simulink model "copied"  (R2019a)
settings: Solver=VariableStepAuto  StartTime=0.0  StopTime=10.0  RelTol=1e-3
libraries: vexarmcortexlib x21, vexcommonlib x3
settings Model: Creator=hsstudent  LastModifiedBy=hsstudent

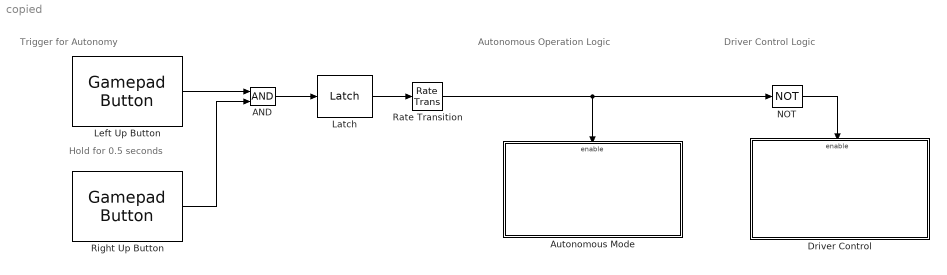
== system copied ==
  note: Autonomous Operation Logic
  note: Trigger for Autonomy
  note: Hold for 0.5 seconds
  note: Driver Control Logic
  AND : Logic  IconShape=distinctive  AllPortsSameDT=off  OutDataTypeStr=boolean
  Autonomous Mode : Subsystem
  Driver Control : Subsystem  TreatAsAtomicUnit=on
  Latch : vexcommonlib/Latch  output0=off  BlockPlatform=vexarmcortex
      settings: SourceProductName=Simulink Coder Support Package for ARM Cortex-based VEX Microcontroller  SourceProductBaseCode=EC_VEX_MICRO
  Left Up Button : vexarmcortexlib/Gamepad/Gamepad Button  joystick=1  chan=7  button56=Down  button78=Up  SimulationIn=off  SampleTime=0.5
      settings: SourceProductName=Simulink Coder Support Package for ARM Cortex-based VEX Microcontroller  SourceProductBaseCode=EC_VEX_MICRO
  NOT : Logic  Operator=NOT  IconShape=distinctive  AllPortsSameDT=off  OutDataTypeStr=boolean
  Rate Transition : RateTransition
  Right Up Button : vexarmcortexlib/Gamepad/Gamepad Button  joystick=1  chan=8  button56=Down  button78=Up  SimulationIn=off  SampleTime=0.5
      settings: SourceProductName=Simulink Coder Support Package for ARM Cortex-based VEX Microcontroller  SourceProductBaseCode=EC_VEX_MICRO
  wires:
  Latch/1 -> Rate Transition/1
  Right Up Button/1 -> AND/2
  Left Up Button/1 -> AND/1
  NOT/1 -> Driver Control/Enable
  Rate Transition/1 -> NOT/1, Autonomous Mode/Enable
  AND/1 -> Latch/1

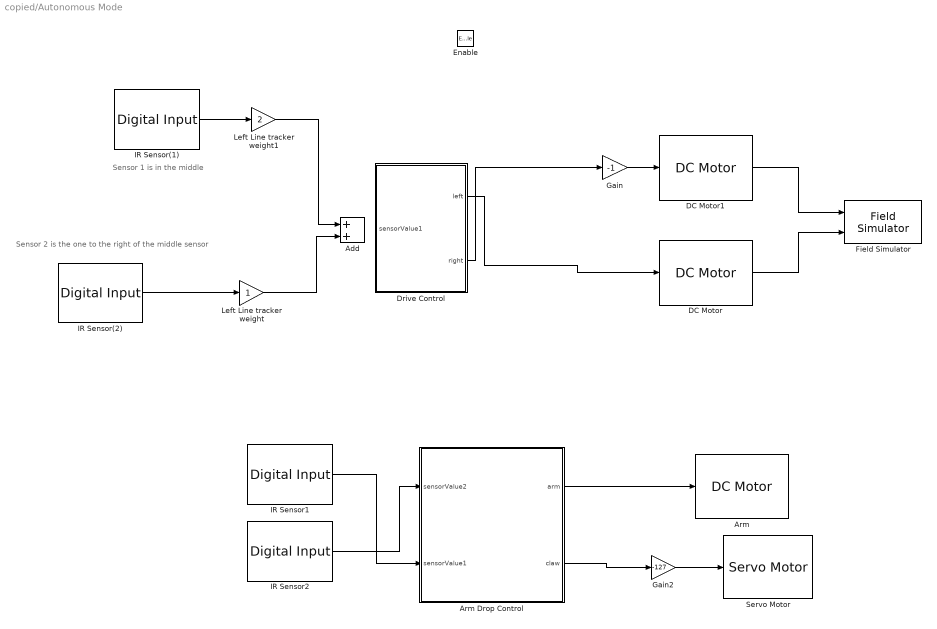
== system copied/Autonomous Mode ==
  note: Sensor 2 is the one to the right of the middle sensor
  note: Sensor 1 is in the middle
  Enable : EnablePort  StatesWhenEnabling=reset
  Add : Sum
  Arm : vexarmcortexlib/Actuators/DC Motor  motor=7  scaleFactor=1/13.5  SimulationOut=on
      settings: SourceProductName=Simulink Coder Support Package for ARM Cortex-based VEX Microcontroller  SourceProductBaseCode=EC_VEX_MICRO
  Arm Drop Control : Stateflow chart  TreatAsAtomicUnit=on
  DC Motor : vexarmcortexlib/Actuators/DC Motor  motor=3  scaleFactor=1/13.5  SimulationOut=on
      settings: SourceProductName=Simulink Coder Support Package for ARM Cortex-based VEX Microcontroller  SourceProductBaseCode=EC_VEX_MICRO
  DC Motor1 : vexarmcortexlib/Actuators/DC Motor  motor=2  scaleFactor=1/13.5  SimulationOut=on
      settings: SourceProductName=Simulink Coder Support Package for ARM Cortex-based VEX Microcontroller  SourceProductBaseCode=EC_VEX_MICRO
  Drive Control : Stateflow chart  TreatAsAtomicUnit=on
  Field Simulator : vexcommonlib/Field Simulator  radius=2.5  space=10  range=200  BlockPlatform=vexarmcortex
      settings: SourceProductName=Simulink Coder Support Package for ARM Cortex-based VEX Microcontroller  SourceProductBaseCode=EC_VEX_MICRO
  Gain : Gain  Gain=-1
  Gain2 : Gain  Gain=-127
  IR Sensor(1) : vexarmcortexlib/Sensors/Digital Input  inChan=9  SimulationIn=off  SampleTime=0.05
      settings: SourceProductName=Simulink Coder Support Package for ARM Cortex-based VEX Microcontroller  SourceProductBaseCode=EC_VEX_MICRO
  IR Sensor(2) : vexarmcortexlib/Sensors/Digital Input  inChan=4  SimulationIn=off  SampleTime=0.05
      settings: SourceProductName=Simulink Coder Support Package for ARM Cortex-based VEX Microcontroller  SourceProductBaseCode=EC_VEX_MICRO
  IR Sensor1 : vexarmcortexlib/Sensors/Digital Input  inChan=9  SimulationIn=off  SampleTime=0.05
      settings: SourceProductName=Simulink Coder Support Package for ARM Cortex-based VEX Microcontroller  SourceProductBaseCode=EC_VEX_MICRO
  IR Sensor2 : vexarmcortexlib/Sensors/Digital Input  inChan=4  SimulationIn=off  SampleTime=0.05
      settings: SourceProductName=Simulink Coder Support Package for ARM Cortex-based VEX Microcontroller  SourceProductBaseCode=EC_VEX_MICRO
  Left Line tracker weight : Gain
  Left Line tracker weight1 : Gain  Gain=2
  Servo Motor : vexarmcortexlib/Actuators/Servo Motor  motor=4  scaleFactor=60/127  SimulationOut=on
      settings: SourceProductName=Simulink Coder Support Package for ARM Cortex-based VEX Microcontroller  SourceProductBaseCode=EC_VEX_MICRO
  wires:
  Gain/1 -> DC Motor1/1
  IR Sensor2/1 -> Arm Drop Control/1(sensorValue2)
  DC Motor1/1 -> Field Simulator/1
  Gain2/1 -> Servo Motor/1
  IR Sensor(2)/1 -> Left Line tracker weight/1
  IR Sensor(1)/1 -> Left Line tracker weight1/1
  Arm Drop Control/2(claw) -> Gain2/1
  DC Motor/1 -> Field Simulator/2
  Drive Control/2(right) -> Gain/1
  IR Sensor1/1 -> Arm Drop Control/2(sensorValue1)
  Drive Control/1(left) -> DC Motor/1
  Arm Drop Control/1(arm) -> Arm/1
  Left Line tracker weight/1 -> Add/2
  Left Line tracker weight1/1 -> Add/1

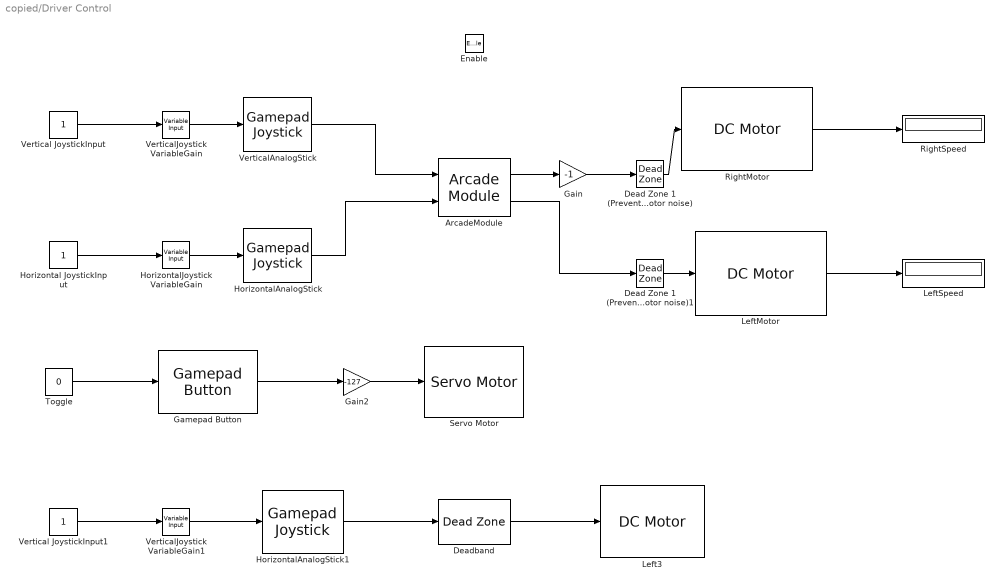
== system copied/Driver Control ==
  Enable : EnablePort  StatesWhenEnabling=reset
  ArcadeModule : vexcommonlib/Arcade Module  BlockPlatform=vexarmcortex
      settings: SourceProductName=Simulink Coder Support Package for ARM Cortex-based VEX Microcontroller  SourceProductBaseCode=EC_VEX_MICRO
  Dead Zone 1 (Prevents motor noise) : DeadZone  LowerValue=-30  UpperValue=30  SaturateOnIntegerOverflow=on
  Dead Zone 1 (Prevents motor noise)1 : DeadZone  LowerValue=-30  UpperValue=30  SaturateOnIntegerOverflow=on
  Deadband : DeadZone  SaturateOnIntegerOverflow=on
  Gain : Gain  Gain=-1
  Gain2 : Gain  Gain=-127
  Gamepad Button : vexarmcortexlib/Gamepad/Gamepad Button  joystick=1  chan=7  button56=Up  button78=Down  SimulationIn=on  SampleTime=0.02
      settings: SourceProductName=Simulink Coder Support Package for ARM Cortex-based VEX Microcontroller  SourceProductBaseCode=EC_VEX_MICRO
  Horizontal JoystickInput : Constant
  HorizontalAnalogStick : vexarmcortexlib/Gamepad/Gamepad Joystick  joystick=1  chan=1  SimulationIn=on  SampleTime=0.02
      settings: SourceProductName=Simulink Coder Support Package for ARM Cortex-based VEX Microcontroller  SourceProductBaseCode=EC_VEX_MICRO
  HorizontalAnalogStick1 : vexarmcortexlib/Gamepad/Gamepad Joystick  joystick=1  chan=3  SimulationIn=on  SampleTime=0.02
      settings: SourceProductName=Simulink Coder Support Package for ARM Cortex-based VEX Microcontroller  SourceProductBaseCode=EC_VEX_MICRO
  HorizontalJoystick VariableGain : vexarmcortexlib/Utilities/Variable Input  low=-127  gain=-118.8065  high=127
      settings: SourceProductName=Simulink Coder Support Package for ARM Cortex-based VEX Microcontroller  SourceProductBaseCode=EC_VEX_MICRO
  Left3 : vexarmcortexlib/Actuators/DC Motor  motor=7  scaleFactor=1/13.5  SimulationOut=on
      settings: SourceProductName=Simulink Coder Support Package for ARM Cortex-based VEX Microcontroller  SourceProductBaseCode=EC_VEX_MICRO
  LeftMotor : vexarmcortexlib/Actuators/DC Motor  motor=3  scaleFactor=1/13.5  SimulationOut=on
      settings: SourceProductName=Simulink Coder Support Package for ARM Cortex-based VEX Microcontroller  SourceProductBaseCode=EC_VEX_MICRO
  LeftSpeed : Display
  RightMotor : vexarmcortexlib/Actuators/DC Motor  motor=2  scaleFactor=1/13.5  SimulationOut=on
      settings: SourceProductName=Simulink Coder Support Package for ARM Cortex-based VEX Microcontroller  SourceProductBaseCode=EC_VEX_MICRO
  RightSpeed : Display
  Servo Motor : vexarmcortexlib/Actuators/Servo Motor  motor=4  scaleFactor=60/127  SimulationOut=on
      settings: SourceProductName=Simulink Coder Support Package for ARM Cortex-based VEX Microcontroller  SourceProductBaseCode=EC_VEX_MICRO
  Toggle : Constant  Value=0
      settings: OpenFcn=|
      | if strcmp('0',get_param(gcb, 'Value'))                        set_param(gcb, 'Value', '1');
      | else
      |             set_param(gcb, 'Value', '0');
      | end
  Vertical JoystickInput : Constant
  Vertical JoystickInput1 : Constant
  VerticalAnalogStick : vexarmcortexlib/Gamepad/Gamepad Joystick  joystick=1  chan=2  SimulationIn=on  SampleTime=0.02
      settings: SourceProductName=Simulink Coder Support Package for ARM Cortex-based VEX Microcontroller  SourceProductBaseCode=EC_VEX_MICRO
  VerticalJoystick VariableGain : vexarmcortexlib/Utilities/Variable Input  low=-127  gain=0  high=127
      settings: SourceProductName=Simulink Coder Support Package for ARM Cortex-based VEX Microcontroller  SourceProductBaseCode=EC_VEX_MICRO
  VerticalJoystick VariableGain1 : vexarmcortexlib/Utilities/Variable Input  low=-127  gain=0  high=127
      settings: SourceProductName=Simulink Coder Support Package for ARM Cortex-based VEX Microcontroller  SourceProductBaseCode=EC_VEX_MICRO
  wires:
  Gain2/1 -> Servo Motor/1
  Toggle/1 -> Gamepad Button/1
  Dead Zone 1 (Prevents motor noise)/1 -> RightMotor/1
  VerticalJoystick VariableGain1/1 -> HorizontalAnalogStick1/1
  Vertical JoystickInput1/1 -> VerticalJoystick VariableGain1/1
  Dead Zone 1 (Prevents motor noise)1/1 -> LeftMotor/1
  HorizontalAnalogStick1/1 -> Deadband/1
  ArcadeModule/1 -> Gain/1
  Vertical JoystickInput/1 -> VerticalJoystick VariableGain/1
  VerticalJoystick VariableGain/1 -> VerticalAnalogStick/1
  RightMotor/1 -> RightSpeed/1
  HorizontalJoystick VariableGain/1 -> HorizontalAnalogStick/1
  LeftMotor/1 -> LeftSpeed/1
  ArcadeModule/2 -> Dead Zone 1 (Prevents motor noise)1/1
  Horizontal JoystickInput/1 -> HorizontalJoystick VariableGain/1
  Gamepad Button/1 -> Gain2/1
  Gain/1 -> Dead Zone 1 (Prevents motor noise)/1
  VerticalAnalogStick/1 -> ArcadeModule/1
  HorizontalAnalogStick/1 -> ArcadeModule/2
  Deadband/1 -> Left3/1

== stateflow chart copied/Autonomous Mode/Arm Drop Control ==
  state Preset
    entry:
    arm = 0;
    claw = 0;
  state TowerDetect
    entry:
    arm = 50;
  state Drop
    entry:
    claw = 1;
    arm = 0;
  state Return
    entry:
    arm = -50;
    claw = 0;
  state Stop
    entry:
    arm = 0;
    claw = 1;
  (default) -> Preset
  TowerDetect -> Drop : after(2,sec)
  Preset -> TowerDetect : [sensorValue1 == 0 || sensorValue2 == 0]
  Drop -> Return
  Return -> Stop : after(2,sec)
  data: sensorValue2 input; sensorValue1 input; arm output; claw output

== stateflow chart copied/Autonomous Mode/Drive Control ==
  state Stop
    entry:
    left = 0;
    right= 0;
  state GoForward
    entry:
    left = 50;
    right = 50;
  state LTurnDetect
    entry:
    right = -50
    left = 50
  state RTurnDetect
    entry:
    right = -50
    left = 50
  (default) -> Stop
  Stop -> GoForward : [sensorValue1 == 0 || sensorValue2 ==1]
  GoForward -> LTurnDetect [order 2] : [sensorValue1 == 1 || sensorValue2 == 1]
  RTurnDetect -> GoForward [order 2] : [sensorValue1 == 0 || sensorValue2 == 1]
  LTurnDetect -> GoForward : [sensorValue1 == 0]
  GoForward -> RTurnDetect [order 1] : [sensorValue1 == 1]
  RTurnDetect -> LTurnDetect [order 1] : [sensorValue1 == 1 || sensorValue2 == 1]
  data: left output; right output; sensorValue1 input
